simulink model "Model_6DOF_2021a"  (R2021b)
settings: Solver=FixedStepAuto  StartTime=0.0  StopTime=Tfin  FixedStep=0.05  RelTol=1e-3
values from neighbouring files (symbols this model uses):
  adap = 1    [ctrl_mode_param.m]
  Ba_0 = [0 0 0 0 0 0]    [ctrl_mode_param.m]
  Bv_0 = [tgt_speed 0 0 0 0 0]    [ctrl_mode_param.m]
  Bx_0 = [0 0 tgt_depth 0 0 0]    [ctrl_mode_param.m]
  check_angle = 10    [ctrl_mode_param.m]
  Cp = [Cpx' ; Cpy' ; Cpz']    [ctrl_mode_param.m]
  Cp_prime = Cp*Dm    [ctrl_mode_param.m]
  ctrl_mode = 5    [run.m]
  dX_imposed = 10    [ctrl_mode_param.m]
  Seastate = 5    [ctrl_mode_param.m]    (also in run.m = 0)
  tgt_depth = -50    [ctrl_mode_param.m]
  tgt_pitch = 0    [ctrl_mode_param.m]
  tgt_speed = -5    [ctrl_mode_param.m]
  tgt_sway = 0    [ctrl_mode_param.m]
  tgt_yaw = 0    [ctrl_mode_param.m]
undefined symbols (not defined in the file or in its folder): Bb, dA_BP1, dA_BP2, dA_Hull, dA_PH, dA_Sail, dA_SProot, dA_X1a, dA_X1b, dA_X2a, dA_X2b, dA_X3a, dA_X3b, dA_X4a, dA_X4b, Ixx, Ixy, Ixz, Iyy, Iyz, Izz, Mb, n_BP1, n_BP2, n_Hull, n_PH, n_Sail, n_SProot, n_X2a, n_X2b, n_X3a, n_X4a, n_X4b, nt_BP1, nt_BP2, nt_Hull, nt_PH, nt_Sail, nt_SProot, nt_X1a, nt_X1b, nt_X2a, nt_X2b, nt_X3a, nt_X3b, nt_X4a, nt_X4b, vt1_BP1, vt1_BP2, vt1_Hull, vt1_PH, vt1_Sail, vt1_SProot, vt1_X1a, vt1_X1b, vt1_X2a, vt1_X2b, vt1_X3a, vt1_X3b, vt1_X4a ... (+36)
libraries: simulink x19
(part 1 of 6)
settings Model: Creator=yagkim  LastModifiedBy=vcichella_l
settings SolverCC: AlgebraicLoopSolver=TrustRegion
settings DebuggingCC: SFMachineParentedDataDiag=warning  ArithmeticOperatorsInVariantConditions=warning
settings SFSimCC: CustomCodeUndefinedFunction=UseInterfaceOnly

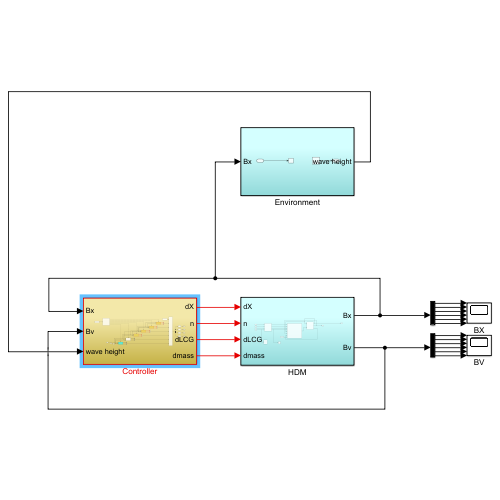
[thumbnail: Simulink's stored preview of the top-level diagram]
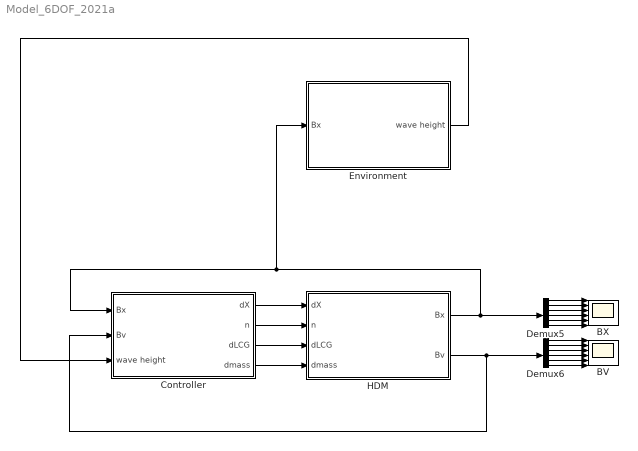
== system Model_6DOF_2021a ==
  BV : Scope  NumInputPorts=6
  BX : Scope  NumInputPorts=6
  Controller : Subsystem
  Demux5 : Demux  Outputs=6
  Demux6 : Demux  Outputs=6
  Environment : Subsystem
  HDM : Subsystem
  wires:
  HDM/1(Bx) -> Environment/1(Bx), Controller/1(Bx), Demux5/1
  Demux6/4 -> BV/4
  HDM/2(Bv) -> Demux6/1, Controller/2(Bv)
  Demux6/6 -> BV/6
  Demux5/5 -> BX/5
  Demux6/2 -> BV/2
  Demux5/6 -> BX/6
  Demux6/5 -> BV/5
  Demux5/4 -> BX/4
  Demux6/1 -> BV/1
  Demux5/3 -> BX/3
  Demux6/3 -> BV/3
  Demux5/2 -> BX/2
  Demux5/1 -> BX/1
  Controller/1(dX) -> HDM/1(dX)
  Controller/2(n) -> HDM/2(n)
  Controller/3(dLCG) -> HDM/3(dLCG)
  Controller/4(dmass) -> HDM/4(dmass)
  Environment/1(wave height) -> Controller/3(wave height)

== system Model_6DOF_2021a/Controller ==
  Bx : Inport
  Bv : Inport  Port=2
  wave height : Inport  Port=3
  Constant : Constant  Value=ctrl_mode
  Constant1 : Constant  Value=ctrl_mode
  HZZ : Subsystem  TreatAsAtomicUnit=on
  Multiport Switch : MultiPortSwitch  Inputs=6
  Mux{,1..5} (6 alike) : Mux
  PF+L1 : Subsystem  TreatAsAtomicUnit=on
  SP : Subsystem  TreatAsAtomicUnit=on
  Selector : Selector  InputPortWidth=8  IndexOptions=Index vector (dialog)  Indices=[1 2 3 4 5]  OutputSizes=1
  Selector1 : Selector  InputPortWidth=8  IndexOptions=Index vector (dialog)  Indices=7  OutputSizes=1
  Selector2 : Selector  InputPortWidth=8  IndexOptions=Index vector (dialog)  Indices=8  OutputSizes=1
  Selector3 : Selector  InputPortWidth=8  IndexOptions=Index vector (dialog)  Indices=6  OutputSizes=1
  Switch Case : SwitchCase  CaseConditions={1,2,3,4,5}
  TC : Subsystem  TreatAsAtomicUnit=on
  VZZ : Subsystem  TreatAsAtomicUnit=on
  customize : Subsystem  TreatAsAtomicUnit=on
  dX : Outport  VectorParamsAs1DForOutWhenUnconnected=off
  n : Outport  Port=2  VectorParamsAs1DForOutWhenUnconnected=off
  dLCG : Outport  Port=3  VectorParamsAs1DForOutWhenUnconnected=off
  dmass : Outport  Port=4  VectorParamsAs1DForOutWhenUnconnected=off
  wires:
  Constant/1 -> Switch Case/1
  Switch Case/1 -> HZZ/Action
  Switch Case/2 -> SP/Action
  Switch Case/3 -> TC/Action
  Switch Case/4 -> VZZ/Action
  Multiport Switch/1 -> Selector3/1, Selector2/1, Selector1/1, Selector/1
  Selector/1 -> dX/1
  Selector3/1 -> n/1
  Selector2/1 -> dmass/1
  Selector1/1 -> dLCG/1
  Bx/1 -> customize/1(Bx), PF+L1/1(Bx), VZZ/1(Bx), HZZ/1(Bx), SP/1(Bx), TC/1(Bx)
  Bv/1 -> customize/2(Bv), PF+L1/2(Bv), VZZ/2(Bv), HZZ/2(Bv), SP/2(Bv), TC/2(Bv)
  HZZ/1(dX) -> Mux/1
  HZZ/2(n) -> Mux/2
  HZZ/3(dLCG) -> Mux/3
  HZZ/4(dmass) -> Mux/4
  SP/1(dX) -> Mux1/1
  SP/2(n) -> Mux1/2
  SP/3(dLCG) -> Mux1/3
  SP/4(dmass) -> Mux1/4
  Mux1/1 -> Multiport Switch/3
  TC/1(dX) -> Mux2/1
  TC/2(n) -> Mux2/2
  TC/3(dLCG) -> Mux2/3
  TC/4(dmass) -> Mux2/4
  VZZ/1(dX) -> Mux3/1
  VZZ/2(n) -> Mux3/2
  VZZ/3(dLCG) -> Mux3/3
  VZZ/4(dmass) -> Mux3/4
  PF+L1/1(dX) -> Mux4/1
  PF+L1/2(n) -> Mux4/2
  PF+L1/3(dLCG) -> Mux4/3
  PF+L1/4(dmass) -> Mux4/4
  Switch Case/5 -> PF+L1/Action
  customize/4(dmass) -> Mux5/4
  customize/3(dLCG) -> Mux5/3
  customize/2(n) -> Mux5/2
  customize/1(dX) -> Mux5/1
  Switch Case/6 -> customize/Action
  wave height/1 -> PF+L1/3(wave height), SP/3(wave height), TC/3(wave height), customize/3(wave height)
  Mux/1 -> Multiport Switch/2
  Mux2/1 -> Multiport Switch/4
  Mux3/1 -> Multiport Switch/5
  Mux4/1 -> Multiport Switch/6
  Mux5/1 -> Multiport Switch/7
  Constant1/1 -> Multiport Switch/1

== system Model_6DOF_2021a/Environment ==
  Bx : Inport
  Constant : Constant  Value=0
  Terminator : Terminator
  wave height : Outport
  wires:
  Bx/1 -> Terminator/1
  Constant/1 -> wave height/1

== system Model_6DOF_2021a/HDM ==
  dX : Inport
  n : Inport  Port=2
  dLCG : Inport  Port=3
  dmass : Inport  Port=4
  Constant1 : Constant  Value=Seastate
  HDM B3 : Subsystem  InitFcn='main'
  Integration and Coord. Transfrom : Subsystem
  Scope : Scope
  Scope1 : Scope
  actuator saturation : Subsystem
  Bx : Outport
  Bv : Outport  Port=2
  wires:
  Integration and Coord. Transfrom/3(Ba) -> HDM B3/7(Ba)
  Integration and Coord. Transfrom/2(Bv) -> Bv/1, HDM B3/6(Bv)
  HDM B3/1(F_hyd) -> Integration and Coord. Transfrom/2(F_hyd)
  Constant1/1 -> HDM B3/8(SeaState)
  Integration and Coord. Transfrom/1("Bx ") -> Bx/1, Integration and Coord. Transfrom/1(Bx), HDM B3/5(Bx)
  dX/1 -> actuator saturation/1("dX ")
  n/1 -> actuator saturation/2("n ")
  dLCG/1 -> actuator saturation/3(dLCG)
  dmass/1 -> Scope/1, actuator saturation/4(dmass)
  actuator saturation/1(dX) -> HDM B3/1(dX CTRL)
  actuator saturation/2(n) -> HDM B3/2(n)
  actuator saturation/3(dLCG (m)) -> HDM B3/3(dLCG)
  actuator saturation/4(dmass (kg)) -> Scope1/1, HDM B3/4(dmass)

== system Model_6DOF_2021a/Controller/HZZ ==
  note: SbDn
  note: SbUp
  note: PsDn
  note: Sail
  note: PsUp
  Bx : Inport
  Bv : Inport  Port=2
  Action Port : ActionPort  ActionPortLabel=case [ 1 ]:
  Add3 : Sum  Inputs=+-
  Add4 : Sum
  Add5 : Sum  Inputs=-+
  Add6 : Sum  Inputs=--
  Constant : Constant  Value=0
  Constant1 : Constant  Value=0
  Constant2 : Constant  Value=tgt_depth
  Gain : Gain  Gain=-1/4
  Gain1 : Gain  Gain=-1
  Mux : Mux  Inputs=5
  Subsystem : Subsystem
  Target Pitch : Constant  Value=tgt_pitch
  Target Speed2 : Constant  Value=tgt_speed
  Terminator : Terminator
  dV PID : Subsystem
  dX : Outport
  n : Outport  Port=2
  dLCG : Outport  Port=3
  dmass : Outport  Port=4
  wires:
  Gain1/1 -> Mux/5
  Add6/1 -> Mux/4
  dV PID/1(dV_pid) -> Add3/1, Add4/1, Add5/1, Add6/1, Gain1/1
  Add4/1 -> Mux/2
  Add3/1 -> Mux/1
  Add5/1 -> Mux/3
  Bx/1 -> dV PID/1(Bx), Subsystem/1(Bx)
  Mux/1 -> dX/1  "dX"
  Target Pitch/1 -> dV PID/2(Target Pitch)
  Constant2/1 -> dV PID/3(Target Height)
  Constant/1 -> dmass/1
  Constant1/1 -> dLCG/1
  Target Speed2/1 -> Gain/1
  Gain/1 -> n/1
  Subsystem/1(dH_HZZ) -> Add3/2, Add6/2, Add5/2, Add4/2
  Bv/1 -> Terminator/1

== system Model_6DOF_2021a/Controller/PF+L1 ==
  Bx : Inport
  Bv : Inport  Port=2
  wave height : Inport  Port=3
  Action Port : ActionPort  ActionPortLabel=case [ 5 ]:
  Constant1 : Constant  Value=0
  Constant2 : Constant  Value=tgt_speed
  Constant3 : Constant  Value=adap
  Scope : Scope
  Stop Simulation : Stop
  Terminator2 : Terminator
  pf_controller : MATLAB Function  TreatAsAtomicUnit=on
  dX : Outport
  n : Outport  Port=2
  dLCG : Outport  Port=3
  dmass : Outport  Port=4
  wires:
  Constant1/1 -> dmass/1, dLCG/1
  wave height/1 -> Terminator2/1
  pf_controller/1(dX) -> dX/1
  pf_controller/2(n) -> n/1
  pf_controller/3(stop) -> Stop Simulation/1
  Constant2/1 -> pf_controller/3(ref)
  Constant3/1 -> pf_controller/4(adap)
  pf_controller/4(pd) -> Scope/1
  Bv/1 -> pf_controller/1(Bv)
  Bx/1 -> pf_controller/2(Bx)

== system Model_6DOF_2021a/Controller/SP ==
  note: PsUp
  note: Sail
  note: PsDn
  note: SbUp
  note: SbDn
  Bx : Inport
  Bv : Inport  Port=2
  wave height : Inport  Port=3
  Action Port : ActionPort  ActionPortLabel=case [ 2 ]:
  " " : Constant  Value=tgt_sway
  "  " : Constant  Value=tgt_yaw
  Add3 : Sum  Inputs=+-
  Add4 : Sum
  Add5 : Sum  Inputs=-+
  Add6 : Sum  Inputs=--
  "Bx " : InportShadow
  Constant : Constant  Value=0
  Gain : Gain  Gain=-1
  Mux : Mux  Inputs=5
  Selector : Selector  InputPortWidth=6  IndexOptions=Index vector (dialog)  Indices=3  OutputSizes=1
  Sum : Sum  Inputs=|+-
  Target Depth2 : Constant  Value=tgt_depth
  Target Height : Constant  Value=tgt_depth
  Target Pitch1 : Constant  Value=tgt_pitch
  Target Pitch2 : Constant  Value=tgt_pitch
  Target Speed1 : Constant  Value=tgt_speed
  Trim and Ballast Tank PID : Subsystem
  dH PID : Subsystem
  dV PID : Subsystem
  n:RPS PID : Subsystem
  dX : Outport
  n : Outport  Port=2
  dLCG : Outport  Port=3
  dmass : Outport  Port=4
  wires:
  n:RPS PID/1(n_ctrl) -> n/1
  Gain/1 -> Mux/5
  Target Speed1/1 -> n:RPS PID/1(Target Speed)
  Target Height/1 -> Trim and Ballast Tank PID/3(Target Height)
  Target Pitch1/1 -> Trim and Ballast Tank PID/2(Target Pitch)
  Mux/1 -> dX/1  "dX"
  "  "/1 -> dH PID/1(Target Yaw)
  " "/1 -> dH PID/2(Target Sway)
  dH PID/1(dH_PID) -> Add4/2, Add6/2, Add5/2, Add3/2
  Bv/1 -> n:RPS PID/2(Bv)
  Add5/1 -> Mux/3
  Add3/1 -> Mux/1
  Add4/1 -> Mux/2
  Add6/1 -> Mux/4
  Constant/1 -> dLCG/1
  "Bx "/1 -> Trim and Ballast Tank PID/1(Bx)
  Selector/1 -> Sum/1  "current"
  Bx/1 -> dH PID/3(Bx), dV PID/1(Bx), Selector/1
  Target Depth2/1 -> dV PID/3(Target Height)
  Target Pitch2/1 -> dV PID/2(Target Pitch)
  dV PID/1(dV_pid) -> Add6/1, Add5/1, Add4/1, Add3/1, Gain/1
  Trim and Ballast Tank PID/2(dmass) -> dmass/1
  wave height/1 -> Sum/2
  Sum/1 -> dV PID/4(Zeff)

== system Model_6DOF_2021a/Controller/TC ==
  note: SbDn
  note: SbUp
  note: PsDn
  note: Sail
  note: PsUp
  Bx : Inport
  Bv : Inport  Port=2
  wave height : Inport  Port=3
  Action Port : ActionPort  ActionPortLabel=case [ 3 ]:
  Add3 : Sum  Inputs=+-
  Add4 : Sum
  Add5 : Sum  Inputs=-+
  Add6 : Sum  Inputs=--
  Bx1 : InportShadow
  Constant : Constant  Value=dX_imposed
  Constant1 : Constant  Value=0
  Gain : Gain  Gain=-1
  Mux : Mux  Inputs=5
  Selector : Selector  InputPortWidth=6  IndexOptions=Index vector (dialog)  Indices=3  OutputSizes=1
  Sum : Sum  Inputs=|+-
  Target Depth1 : Constant  Value=tgt_depth
  Target Height : Constant  Value=tgt_depth
  Target Pitch : Constant  Value=tgt_pitch
  Target Pitch1 : Constant  Value=tgt_pitch
  Target Speed1 : Constant  Value=tgt_speed
  Trim and Ballast Tank PID : Subsystem
  dV PID : Subsystem
  n:RPS PID : Subsystem
  dX : Outport
  n : Outport  Port=2
  dLCG : Outport  Port=3
  dmass : Outport  Port=4
  wires:
  Gain/1 -> Mux/5
  Add6/1 -> Mux/4
  dV PID/1(dV_pid) -> Add3/1, Add4/1, Add5/1, Add6/1, Gain/1
  Add4/1 -> Mux/2
  Add3/1 -> Mux/1
  Add5/1 -> Mux/3
  Bv/1 -> n:RPS PID/2(Bv)
  Mux/1 -> dX/1  "dX"
  n:RPS PID/1(n_ctrl) -> n/1
  Target Pitch/1 -> dV PID/2(Target Pitch)
  Target Speed1/1 -> n:RPS PID/1(Target Speed)
  Target Depth1/1 -> dV PID/3(Target Height)
  Constant/1 -> Add6/2, Add5/2, Add4/2, Add3/2
  Constant1/1 -> dLCG/1
  Trim and Ballast Tank PID/2(dmass) -> dmass/1
  Target Pitch1/1 -> Trim and Ballast Tank PID/2(Target Pitch)
  Target Height/1 -> Trim and Ballast Tank PID/3(Target Height)
  Bx1/1 -> Trim and Ballast Tank PID/1(Bx)
  Selector/1 -> Sum/1  "current"
  Bx/1 -> Selector/1, dV PID/1(Bx)
  wave height/1 -> Sum/2
  Sum/1 -> dV PID/4(Zeff)

== system Model_6DOF_2021a/Controller/VZZ ==
  note: PsUp
  note: Sail
  note: PsDn
  note: SbUp
  note: SbDn
  Bx : Inport
  Bv : Inport  Port=2
  Action Port : ActionPort  ActionPortLabel=case [ 4 ]:
  " " : Constant  Value=tgt_sway
  "  " : Constant  Value=tgt_yaw
  Add3 : Sum  Inputs=+-
  Add4 : Sum
  Add5 : Sum  Inputs=-+
  Add6 : Sum  Inputs=--
  Constant : Constant  Value=0
  Constant1 : Constant  Value=0
  Constant2 : Constant  Value=0
  Gain : Gain  Gain=-1/4
  Gain2 : Gain  Gain=-1
  Mux : Mux  Inputs=5
  Scope : Scope
  Target Speed2 : Constant  Value=tgt_speed
  Terminator : Terminator
  dH PID : Subsystem
  dV : Subsystem
  dX : Outport
  n : Outport  Port=2
  dLCG : Outport  Port=3
  dmass : Outport  Port=4
  wires:
  Gain2/1 -> Mux/5
  Mux/1 -> dX/1  "dX"
  "  "/1 -> dH PID/1(Target Yaw)
  " "/1 -> dH PID/2(Target Sway)
  dH PID/1(dH_PID) -> Add4/2, Add6/2, Add5/2, Add3/2
  Bx/1 -> dH PID/3(Bx), dV/1(Bx)
  Add5/1 -> Mux/3
  Add3/1 -> Mux/1
  Add4/1 -> Mux/2
  Add6/1 -> Mux/4
  Target Speed2/1 -> Gain/1
  Gain/1 -> n/1
  Constant1/1 -> dLCG/1
  Constant/1 -> dmass/1
  dV/1(dV_VZZ) -> Scope/1, Add6/1, Add5/1, Add4/1, Add3/1
  Bv/1 -> Terminator/1
  Constant2/1 -> Gain2/1

== system Model_6DOF_2021a/Controller/customize ==
  Bx : Inport
  Bv : Inport  Port=2
  wave height : Inport  Port=3
  Action Port : ActionPort  ActionPortLabel=default:
  Constant : Constant  Value=zeros(5,1)
  Constant1 : Constant  Value=0
  Terminator : Terminator
  Terminator1 : Terminator
  Terminator2 : Terminator
  dX : Outport
  n : Outport  Port=2
  dLCG : Outport  Port=3
  dmass : Outport  Port=4
  wires:
  Constant1/1 -> dmass/1, n/1, dLCG/1
  Constant/1 -> dX/1
  Bv/1 -> Terminator1/1
  Bx/1 -> Terminator/1
  wave height/1 -> Terminator2/1

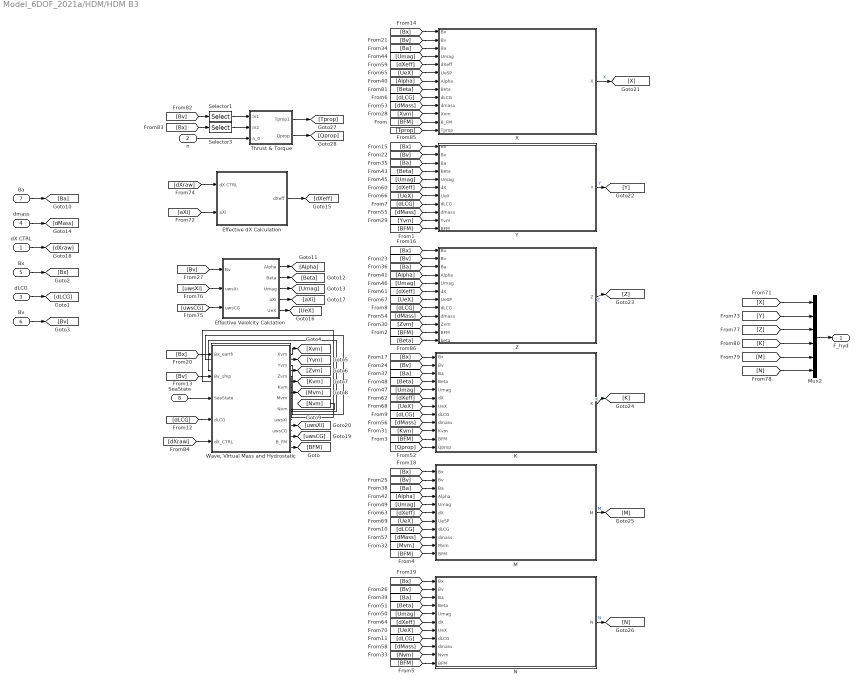
== system Model_6DOF_2021a/HDM/HDM B3 ==
  dX CTRL : Inport
  n : Inport  Port=2
  dLCG : Inport  Port=3
  dmass : Inport  Port=4
  Bx : Inport  Port=5
  Bv : Inport  Port=6
  Ba : Inport  Port=7
  SeaState : Inport  Port=8
  Effective Veloicity Calclation : Subsystem
  Effective dX Calculation : Subsystem
  K : Subsystem
  M : Subsystem
  Mux2 : Mux  Inputs=6
  N : Subsystem
  Selector1 : Selector  InputPortWidth=6  IndexOptions=Index vector (dialog)  Indices=1  OutputSizes=1
  Selector3 : Selector  InputPortWidth=6  IndexOptions=Index vector (dialog)  Indices=3  OutputSizes=1
  Thrust & Torque : Subsystem
  "Wave, Virtual Mass and Hydrostatic" : Subsystem
  X : Subsystem
  Y : Subsystem
  Z : Subsystem
  F_hyd : Outport  VectorParamsAs1DForOutWhenUnconnected=off
  wires:
  Mux2/1 -> F_hyd/1
  Effective dX Calculation/1(dXeff) -> [dXeff]
  Ba/1 -> [Ba]
  Bx/1 -> [Bx]
  dLCG/1 -> [dLCG]
  Bv/1 -> [Bv]
  SeaState/1 -> "Wave, Virtual Mass and Hydrostatic"/3(SeaState)
  n/1 -> Thrust & Torque/3(n_0)
  "Wave, Virtual Mass and Hydrostatic"/9(B_FM) -> [BFM]
  [BFM] -> X/12(B_FM)
  [BFM] -> Y/11(BFM)
  [BFM] -> Z/11(BFM)
  [BFM] -> K/11(BFM)
  [BFM] -> M/11(BFM)
  [BFM] -> N/11(BFM)
  [dLCG] -> X/9(dLCG)
  [dLCG] -> Y/8(dLCG)
  [dLCG] -> Z/8(dLCG)
  [dLCG] -> K/8(dLCG)
  [dLCG] -> M/8(dLCG)
  [dLCG] -> N/8(dLCG)
  [dLCG] -> "Wave, Virtual Mass and Hydrostatic"/4(dLCG)
  [Bx] -> X/1(Bx)
  [Bx] -> Y/1(Bx)
  [Bx] -> Z/1(Bx)
  [Bx] -> K/1(Bx)
  [Bx] -> M/1(Bx)
  [Bx] -> N/1(Bx)
  [Bx] -> "Wave, Virtual Mass and Hydrostatic"/1(Bx_earth)
  [Bv] -> "Wave, Virtual Mass and Hydrostatic"/2(Bv_ship)
  [Bv] -> X/2(Bv)
  [Bv] -> Y/2(Bv)
  [Bv] -> K/2(Bv)
  [Bv] -> M/2(Bv)
  [Bv] -> N/2(Bv)
  [Bv] -> Effective Veloicity Calclation/1(Bv)
  "Wave, Virtual Mass and Hydrostatic"/1(Xvm) -> [Xvm]
  "Wave, Virtual Mass and Hydrostatic"/2(Yvm) -> [Yvm]
  "Wave, Virtual Mass and Hydrostatic"/3(Zvm) -> [Zvm]
  "Wave, Virtual Mass and Hydrostatic"/4(Kvm) -> [Kvm]
  "Wave, Virtual Mass and Hydrostatic"/5(Mvm) -> [Mvm]
  "Wave, Virtual Mass and Hydrostatic"/6(Nvm) -> [Nvm]
  [Xvm] -> X/11(Xvm)
  [Yvm] -> Y/10(Yvm)
  [Zvm] -> Z/10(Zvm)
  [Bv] -> Z/2(Bv)
  [Kvm] -> K/10(Kvm)
  [Mvm] -> M/10(Mvm)
  [Nvm] -> N/10(Nvm)
  [Ba] -> X/3(Ba)
  [Ba] -> Y/3(Ba)
  [Ba] -> Z/3(Ba)
  [Ba] -> K/3(Ba)
  [Ba] -> M/3(Ba)
  [Ba] -> N/3(Ba)
  Effective Veloicity Calclation/1(Alpha) -> [Alpha]
  [Alpha] -> X/7(Alpha)
  [Alpha] -> Z/4(Alpha)
  [Alpha] -> M/4(Alpha)
  Effective Veloicity Calclation/2(Beta) -> [Beta]
  [Beta] -> Y/4(Beta)
  Effective Veloicity Calclation/3(Umag) -> [Umag]
  [Umag] -> X/4(Umag)
  [Umag] -> Y/5(Umag)
  [Umag] -> Z/5(Umag)
  [Umag] -> K/5(Umag)
  [Beta] -> K/4(Beta)
  [Umag] -> M/5(Umag)
  [Umag] -> N/5(Umag)
  [Beta] -> N/4(Beta)
  dmass/1 -> [dMass]
  [dMass] -> X/10(dmass)
  [dMass] -> Z/9(dmass)
  [dMass] -> Y/9(dmass)
  [dMass] -> K/9(dmass)
  [dMass] -> M/9(dmass)
  [dMass] -> N/9(dmass)
  [dXeff] -> X/5(dXeff)
  [dXeff] -> Y/6(dX)
  [dXeff] -> Z/6(dX)
  [dXeff] -> K/6(dX)
  [dXeff] -> M/6(dX)
  [dXeff] -> N/6(dX)
  Effective Veloicity Calclation/5(UeX) -> [UeX]
  [UeX] -> X/6(UeSP)
  [UeX] -> Y/7(UeX)
  [UeX] -> Z/7(UeSP)
  [UeX] -> K/7(UeX)
  [UeX] -> M/7(UeSP)
  [UeX] -> N/7(UeX)
  Effective Veloicity Calclation/4(aXi) -> [aXi]
  [aXi] -> Effective dX Calculation/2(aXi)
  dX CTRL/1 -> [dXraw]
  [dXraw] -> Effective dX Calculation/1(dX CTRL)
  "Wave, Virtual Mass and Hydrostatic"/8(uwsCG) -> [uwsCG]
  [uwsCG] -> Effective Veloicity Calclation/3(uwsCG)
  "Wave, Virtual Mass and Hydrostatic"/7(uwsXi) -> [uwsXi]
  [uwsXi] -> Effective Veloicity Calclation/2(uwsXi)
  X/1(X) -> [X]  "X"
  Y/1(Y) -> [Y]  "Y"
  Z/1(Z) -> [Z]  "Z"
  K/1(K) -> [K]  "K"
  M/1(M) -> [M]  "M"
  N/1(N) -> [N]  "N"
  [Beta] -> X/8(Beta)
  [dXraw] -> "Wave, Virtual Mass and Hydrostatic"/5(dX_CTRL)
  [X] -> Mux2/1
  [Y] -> Mux2/2
  [Z] -> Mux2/3
  [K] -> Mux2/4
  [M] -> Mux2/5
  [N] -> Mux2/6
  [Qprop] -> K/12(Qprop)
  [Bv] -> Selector1/1
  Selector1/1 -> Thrust & Torque/1(In1)
  Selector3/1 -> Thrust & Torque/2(In2)
  [Bx] -> Selector3/1
  Thrust & Torque/1(Tprop1) -> [Tprop]
  [Tprop] -> X/13(Tprop)
  Thrust & Torque/2(Qprop) -> [Qprop]
  [Beta] -> Z/12(beta)

== system Model_6DOF_2021a/HDM/Integration and Coord. Transfrom ==
  Bx : Inport
  F_hyd : Inport  Port=2
  Coordinate Transform : Subsystem
  Rigid Body Motion : Subsystem
  "Bx " : Outport
  Bv : Outport  Port=2
  Ba : Outport  Port=3
  wires:
  Coordinate Transform/1(X_earth) -> "Bx "/1
  Rigid Body Motion/1(Bv) -> Bv/1, Coordinate Transform/1(Bv)
  Rigid Body Motion/2(Ba) -> Ba/1
  F_hyd/1 -> Rigid Body Motion/1(F_hyd)
  Bx/1 -> Rigid Body Motion/2(Bx)

== system Model_6DOF_2021a/HDM/actuator saturation ==
  "dX " : Inport
  "n " : Inport  Port=2
  dLCG : Inport  Port=3
  dmass : Inport  Port=4
  " " : Subsystem
  "   " : Subsystem
  Subsystem1 : Subsystem
  Subsystem2 : Subsystem
  dX : Outport
  n : Outport  Port=2
  dLCG (m) : Outport  Port=3
  dmass (kg) : Outport  Port=4
  wires:
  "   "/1(n) -> n/1
  " "/1(dX) -> dX/1
  dLCG/1 -> Subsystem1/1(dLCG)
  Subsystem1/1(dLCG (m)) -> dLCG (m)/1
  dmass/1 -> Subsystem2/1(dmass)
  "dX "/1 -> " "/1("dX ")
  Subsystem2/1(dmass (kg)) -> dmass (kg)/1
  "n "/1 -> "   "/1("n ")

== system Model_6DOF_2021a/Controller/HZZ/Subsystem ==
  Bx : Inport
  Clock : Clock
  Constant4 : Constant  Value=dX_imposed
  Constant6 : Constant  Value=check_angle
  Gain1 : Gain  Gain=-1
  Gain10 : Gain  Gain=180/pi
  Integrator2 : Integrator
  MATLAB Function : MATLAB Function  TreatAsAtomicUnit=on
  Max Fin Rate : Constant  Value=7.11
  Saturation1 : Saturate  UpperLimit=20  LowerLimit=-20
  Selector3 : Selector  InputPortWidth=6  IndexOptions=Index vector (dialog)  Indices=6  OutputSizes=1
  dH_HZZ : Outport
  wires:
  Saturation1/1 -> MATLAB Function/4(dVprev), Gain1/1
  Bx/1 -> Selector3/1
  Selector3/1 -> Gain10/1
  Max Fin Rate/1 -> MATLAB Function/1(rate)
  Clock/1 -> MATLAB Function/2(trigger)
  Gain10/1 -> MATLAB Function/3(X5)
  MATLAB Function/1(dVrate) -> Integrator2/1
  Integrator2/1 -> Saturation1/1
  Constant6/1 -> MATLAB Function/6(dXmax)
  Constant4/1 -> MATLAB Function/5(dVmax)
  Gain1/1 -> dH_HZZ/1

== system Model_6DOF_2021a/Controller/HZZ/dV PID ==
  Bx : Inport
  Target Pitch : Inport  Port=2
  Target Height : Inport  Port=3
  Add : Sum  Inputs=+++
  Add1 : Sum  Inputs=+++
  Add10 : Sum
  Add7 : Sum  Inputs=-+
  Add9 : Sum  Inputs=-+
  Constant : Constant  Value=7.11
  Constant1 : Constant  Value=-7.11
  D-Depth : Gain  Gain=3
  D-Pitch : Gain  Gain=3
  Derivative : Derivative
  Derivative3 : Derivative
  Gain36 : Gain  Gain=180/pi
  I-Depth : Gain  Gain=0.1044
  I-Pitch : Gain  Gain=0.1466
  I-Pitch{1..6} (6 alike) : Gain
  Integrator : Integrator
  Integrator3 : Integrator
  Max Deflection1 : Saturate  UpperLimit=30  LowerLimit=-30
  P-Depth : Gain  Gain=3
  P-Pitch : Gain  Gain=3
  PID Pitch : Selector  InputPortWidth=6  IndexOptions=Index vector (dialog)  Indices=5  OutputSizes=1
  PID Pitch1 : Selector  InputPortWidth=6  IndexOptions=Index vector (dialog)  Indices=3  OutputSizes=1
  Rate Limiter Dynamic : simulink/Discontinuities/Rate Limiter Dynamic
  dV_pid : Outport
  wires:
  Max Deflection1/1 -> dV_pid/1  "dV"
  Add/1 -> Add10/2  "dV Depth (deg)"
  Add7/1 -> Derivative3/1, Integrator/1, P-Depth/1  "Erorr in z (m)"
  PID Pitch1/1 -> Add7/2  "z (m)"
  Integrator/1 -> I-Depth/1
  P-Depth/1 -> I-Pitch4/1
  Gain36/1 -> Add9/2  "Pitch (deg)"
  Add9/1 -> Derivative/1, Integrator3/1, P-Pitch/1  "Error in Pitch (deg)"
  P-Pitch/1 -> I-Pitch3/1
  Bx/1 -> PID Pitch1/1, PID Pitch/1
  Derivative3/1 -> D-Depth/1
  Add1/1 -> Add10/1  "dV Pitch (deg)"
  D-Depth/1 -> I-Pitch6/1
  Derivative/1 -> D-Pitch/1
  Integrator3/1 -> I-Pitch/1
  PID Pitch/1 -> Gain36/1
  Rate Limiter Dynamic/1 -> Max Deflection1/1  "dV"
  D-Pitch/1 -> I-Pitch5/1
  Target Pitch/1 -> Add9/1
  Add10/1 -> Rate Limiter Dynamic/2
  Constant/1 -> Rate Limiter Dynamic/1
  Constant1/1 -> Rate Limiter Dynamic/3
  Target Height/1 -> Add7/1
  I-Pitch/1 -> I-Pitch1/1
  I-Depth/1 -> I-Pitch2/1
  I-Pitch1/1 -> Add1/2
  I-Pitch2/1 -> Add/2
  I-Pitch3/1 -> Add1/1
  I-Pitch4/1 -> Add/1
  I-Pitch5/1 -> Add1/3
  I-Pitch6/1 -> Add/3

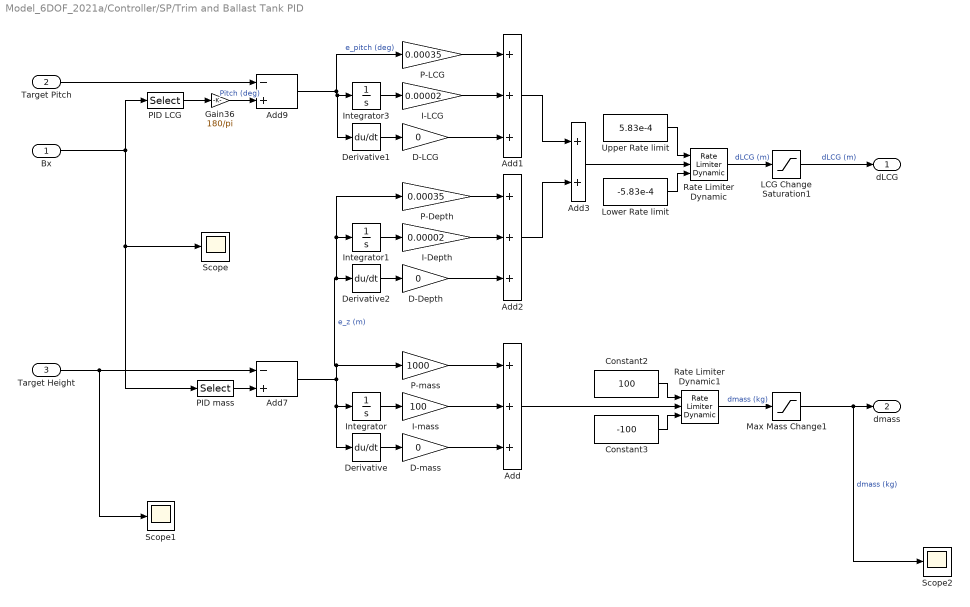
== system Model_6DOF_2021a/Controller/SP/Trim and Ballast Tank PID ==
  Bx : Inport
  Target Pitch : Inport  Port=2
  Target Height : Inport  Port=3
  " LCG Change Saturation1" : Saturate
  Add : Sum  Inputs=+++
  Add1 : Sum  Inputs=+++
  Add2 : Sum  Inputs=+++
  Add3 : Sum
  Add7 : Sum  Inputs=-+
  Add9 : Sum  Inputs=-+
  Constant2 : Constant  Value=100
  Constant3 : Constant  Value=-100
  D-Depth : Gain  Gain=0
  D-LCG : Gain  Gain=0
  D-mass : Gain  Gain=0
  Derivative : Derivative
  Derivative1 : Derivative
  Derivative2 : Derivative
  Gain36 : Gain  Gain=180/pi
  I-Depth : Gain  Gain=0.00002
  I-LCG : Gain  Gain=0.00002
  I-mass : Gain  Gain=100
  Integrator : Integrator
  Integrator1 : Integrator
  Integrator3 : Integrator
  Lower Rate limit : Constant  Value=-5.83e-4
  Max Mass Change1 : Saturate  UpperLimit=20000  LowerLimit=-20000
  P-Depth : Gain  Gain=0.00035
  P-LCG : Gain  Gain=0.00035
  P-mass : Gain  Gain=1000
  PID LCG : Selector  InputPortWidth=6  IndexOptions=Index vector (dialog)  Indices=5  OutputSizes=1
  PID mass : Selector  InputPortWidth=6  IndexOptions=Index vector (dialog)  Indices=3  OutputSizes=1
  Rate Limiter Dynamic : simulink/Discontinuities/Rate Limiter Dynamic
  Rate Limiter Dynamic1 : simulink/Discontinuities/Rate Limiter Dynamic
  Scope : Scope
  Scope1 : Scope
  Scope2 : Scope
  Upper Rate limit : Constant  Value=5.83e-4
  dLCG : Outport
  dmass : Outport  Port=2
  wires:
  " LCG Change Saturation1"/1 -> dLCG/1  "dLCG (m)"
  Max Mass Change1/1 -> Scope2/1, dmass/1  "dmass (kg)"
  Add9/1 -> P-LCG/1, Integrator3/1, Derivative1/1  "e_pitch (deg)"
  Add7/1 -> P-mass/1, Derivative2/1, Integrator1/1, P-Depth/1, Integrator/1, Derivative/1  "e_z (m)"
  Add2/1 -> Add3/2
  Add1/1 -> Add3/1
  Add3/1 -> Rate Limiter Dynamic/2
  P-Depth/1 -> Add2/1
  D-Depth/1 -> Add2/3
  Derivative2/1 -> D-Depth/1
  Integrator1/1 -> I-Depth/1
  I-Depth/1 -> Add2/2
  Constant3/1 -> Rate Limiter Dynamic1/3
  Constant2/1 -> Rate Limiter Dynamic1/1
  Add/1 -> Rate Limiter Dynamic1/2
  Rate Limiter Dynamic1/1 -> Max Mass Change1/1  "dmass (kg)"
  Lower Rate limit/1 -> Rate Limiter Dynamic/3
  Upper Rate limit/1 -> Rate Limiter Dynamic/1
  Target Pitch/1 -> Add9/1
  P-mass/1 -> Add/1
  I-LCG/1 -> Add1/2
  Integrator3/1 -> I-LCG/1
  Derivative1/1 -> D-LCG/1
  PID mass/1 -> Add7/2
  Derivative/1 -> D-mass/1
  Target Height/1 -> Scope1/1, Add7/1
  Integrator/1 -> I-mass/1
  Rate Limiter Dynamic/1 -> " LCG Change Saturation1"/1  "dLCG (m)"
  PID LCG/1 -> Gain36/1
  D-LCG/1 -> Add1/3
  P-LCG/1 -> Add1/1
  Gain36/1 -> Add9/2  "Pitch (deg)"
  I-mass/1 -> Add/2
  Bx/1 -> Scope/1, PID mass/1, PID LCG/1
  D-mass/1 -> Add/3

== system Model_6DOF_2021a/Controller/SP/dH PID ==
  Target Yaw : Inport
  Target Sway : Inport  Port=2
  Bx : Inport  Port=3
  Add1 : Sum  Inputs=+++
  Add10 : Sum
  Add2 : Sum  Inputs=+++
  Add7 : Sum  Inputs=-+
  Add9 : Sum  Inputs=-+
  Constant : Constant  Value=7.11
  Constant1 : Constant  Value=-7.11
  D-Sway : Gain  Gain=0
  D-Yaw : Gain  Gain=12.199
  Derivative : Derivative
  Derivative1 : Derivative
  Gain36 : Gain  Gain=180/pi
  I-Sway : Gain  Gain=0
  I-Yaw : Gain  Gain=0
  Integrator : Integrator
  Integrator3 : Integrator
  Max Deflection : Saturate  UpperLimit=30  LowerLimit=-30
  P-Sway1 : Gain  Gain=-1.452
  P-Yaw : Gain  Gain=3
  PID Sway : Selector  InputPortWidth=6  IndexOptions=Index vector (dialog)  Indices=2  OutputSizes=1
  PID Yaw : Selector  InputPortWidth=6  IndexOptions=Index vector (dialog)  Indices=6  OutputSizes=1
  Rate Limiter Dynamic : simulink/Discontinuities/Rate Limiter Dynamic
  dH_PID : Outport
  wires:
  Max Deflection/1 -> dH_PID/1
  Constant/1 -> Rate Limiter Dynamic/1
  Constant1/1 -> Rate Limiter Dynamic/3
  Target Yaw/1 -> Add9/1
  Add10/1 -> Rate Limiter Dynamic/2
  Derivative1/1 -> D-Yaw/1
  D-Sway/1 -> Add2/3
  P-Sway1/1 -> Add2/1
  Rate Limiter Dynamic/1 -> Max Deflection/1
  Gain36/1 -> Add9/2
  Integrator/1 -> I-Sway/1
  Add1/1 -> Add10/1
  PID Yaw/1 -> Gain36/1
  D-Yaw/1 -> Add1/3
  I-Sway/1 -> Add2/2
  Bx/1 -> PID Sway/1, PID Yaw/1
  P-Yaw/1 -> Add1/1
  PID Sway/1 -> Add7/2
  Derivative/1 -> D-Sway/1
  Target Sway/1 -> Add7/1
  Add7/1 -> Integrator/1, Derivative/1, P-Sway1/1
  I-Yaw/1 -> Add1/2
  Add2/1 -> Add10/2
  Add9/1 -> Integrator3/1, Derivative1/1, P-Yaw/1
  Integrator3/1 -> I-Yaw/1

== system Model_6DOF_2021a/Controller/SP/dV PID ==
  Bx : Inport
  Target Pitch : Inport  Port=2
  Target Height : Inport  Port=3
  Zeff : Inport  Port=4
  Add : Sum  Inputs=+++
  Add1 : Sum  Inputs=+++
  Add10 : Sum
  Add7 : Sum  Inputs=-+
  Add9 : Sum  Inputs=-+
  Constant : Constant  Value=7.11
  Constant1 : Constant  Value=-7.11
  D-Depth : Gain  Gain=3
  D-Pitch : Gain  Gain=3
  Derivative : Derivative
  Derivative3 : Derivative
  Gain36 : Gain  Gain=180/pi
  I-Depth : Gain  Gain=0.1044
  I-Pitch : Gain  Gain=0.1466
  I-Pitch{1..6} (6 alike) : Gain
  Integrator : Integrator
  Integrator3 : Integrator
  Max Deflection1 : Saturate  UpperLimit=30  LowerLimit=-30
  P-Depth : Gain  Gain=3
  P-Pitch : Gain  Gain=3
  PID Pitch : Selector  InputPortWidth=6  IndexOptions=Index vector (dialog)  Indices=5  OutputSizes=1
  Rate Limiter Dynamic : simulink/Discontinuities/Rate Limiter Dynamic
  dV_pid : Outport
  wires:
  Max Deflection1/1 -> dV_pid/1  "dV"
  Add/1 -> Add10/2  "dV Depth (deg)"
  Add7/1 -> Derivative3/1, Integrator/1, P-Depth/1  "Erorr in z (m)"
  Zeff/1 -> Add7/2  "z (m)"
  Integrator/1 -> I-Depth/1
  P-Depth/1 -> I-Pitch4/1
  Gain36/1 -> Add9/2  "Pitch (deg)"
  Add9/1 -> Derivative/1, Integrator3/1, P-Pitch/1  "Error in Pitch (deg)"
  P-Pitch/1 -> I-Pitch3/1
  Bx/1 -> PID Pitch/1
  Derivative3/1 -> D-Depth/1
  Add1/1 -> Add10/1  "dV Pitch (deg)"
  D-Depth/1 -> I-Pitch6/1
  Derivative/1 -> D-Pitch/1
  Integrator3/1 -> I-Pitch/1
  PID Pitch/1 -> Gain36/1
  Rate Limiter Dynamic/1 -> Max Deflection1/1  "dV"
  D-Pitch/1 -> I-Pitch5/1
  Target Pitch/1 -> Add9/1
  Add10/1 -> Rate Limiter Dynamic/2
  Constant/1 -> Rate Limiter Dynamic/1
  Constant1/1 -> Rate Limiter Dynamic/3
  Target Height/1 -> Add7/1
  I-Pitch/1 -> I-Pitch1/1
  I-Depth/1 -> I-Pitch2/1
  I-Pitch1/1 -> Add1/2
  I-Pitch2/1 -> Add/2
  I-Pitch3/1 -> Add1/1
  I-Pitch4/1 -> Add/1
  I-Pitch5/1 -> Add1/3
  I-Pitch6/1 -> Add/3

== system Model_6DOF_2021a/Controller/SP/n:RPS PID ==
  Target Speed : Inport
  Bv : Inport  Port=2
  Add : Sum  Inputs=+++
  Add1 : Sum  Inputs=-+
  Constant1 : Constant  Value=4
  Divide : Product  Inputs=*/
  Gain1 : Gain  Gain=14.65
  Gain4 : Gain  Gain=1.465
  Integrator : Integrator
  Rate Limiter Dynamic : simulink/Discontinuities/Rate Limiter Dynamic
  Rate Max : Constant  Value=14.65
  Rate Min : Constant  Value=-14.65
  Saturation1 : Saturate  UpperLimit=10  LowerLimit=0.01
  Selector : Selector  InputPortWidth=6  IndexOptions=Index vector (dialog)  Indices=1  OutputSizes=1
  n_ctrl : Outport  VectorParamsAs1DForOutWhenUnconnected=off
  wires:
  Saturation1/1 -> n_ctrl/1
  Rate Limiter Dynamic/1 -> Saturation1/1
  Integrator/1 -> Gain4/1
  Rate Min/1 -> Rate Limiter Dynamic/3
  Rate Max/1 -> Rate Limiter Dynamic/1
  Divide/1 -> Add/1
  Add/1 -> Rate Limiter Dynamic/2
  Gain1/1 -> Add/2
  Gain4/1 -> Add/3
  Bv/1 -> Selector/1
  Add1/1 -> Integrator/1, Gain1/1  "error term"
  Target Speed/1 -> Divide/1, Add1/1  "target"
  Constant1/1 -> Divide/2
  Selector/1 -> Add1/2  "current"

== system Model_6DOF_2021a/Controller/TC/Trim and Ballast Tank PID ==
  Bx : Inport
  Target Pitch : Inport  Port=2
  Target Height : Inport  Port=3
  " LCG Change Saturation" : Saturate
  Add : Sum  Inputs=+++
  Add1 : Sum  Inputs=+++
  Add2 : Sum  Inputs=+++
  Add3 : Sum
  Add7 : Sum  Inputs=-+
  Add9 : Sum  Inputs=-+
  Constant2 : Constant  Value=100
  Constant3 : Constant  Value=-100
  D-Depth : Gain  Gain=0
  D-LCG : Gain  Gain=0
  D-mass : Gain  Gain=0
  Derivative : Derivative
  Derivative1 : Derivative
  Derivative2 : Derivative
  Gain36 : Gain  Gain=180/pi
  I-Depth : Gain  Gain=0.00002
  I-LCG : Gain  Gain=0.00002
  I-mass : Gain  Gain=100
  Integrator : Integrator
  Integrator1 : Integrator
  Integrator3 : Integrator
  Lower Rate limit : Constant  Value=-5.83e-4
  Max Mass Change : Saturate  UpperLimit=20000  LowerLimit=-20000
  P-Depth : Gain  Gain=0.00035
  P-LCG : Gain  Gain=0.00035
  P-mass : Gain  Gain=1000
  PID LCG : Selector  InputPortWidth=6  IndexOptions=Index vector (dialog)  Indices=5  OutputSizes=1
  PID mass : Selector  InputPortWidth=6  IndexOptions=Index vector (dialog)  Indices=3  OutputSizes=1
  Rate Limiter Dynamic : simulink/Discontinuities/Rate Limiter Dynamic
  Rate Limiter Dynamic1 : simulink/Discontinuities/Rate Limiter Dynamic
  Upper Rate limit : Constant  Value=5.83e-4
  dLCG : Outport
  dmass : Outport  Port=2
  wires:
  " LCG Change Saturation"/1 -> dLCG/1  "dLCG (m)"
  Max Mass Change/1 -> dmass/1  "dmass (kg)"
  D-mass/1 -> Add/3
  Bx/1 -> PID LCG/1, PID mass/1
  I-mass/1 -> Add/2
  Gain36/1 -> Add9/2  "Pitch (deg)"
  P-LCG/1 -> Add1/1
  D-LCG/1 -> Add1/3
  PID LCG/1 -> Gain36/1
  Rate Limiter Dynamic/1 -> " LCG Change Saturation"/1
  Integrator/1 -> I-mass/1
  Target Height/1 -> Add7/1
  Derivative/1 -> D-mass/1
  PID mass/1 -> Add7/2
  Derivative1/1 -> D-LCG/1
  Integrator3/1 -> I-LCG/1
  I-LCG/1 -> Add1/2
  P-mass/1 -> Add/1
  Target Pitch/1 -> Add9/1
  Upper Rate limit/1 -> Rate Limiter Dynamic/1
  Lower Rate limit/1 -> Rate Limiter Dynamic/3
  Add/1 -> Rate Limiter Dynamic1/2
  Rate Limiter Dynamic1/1 -> Max Mass Change/1
  Constant2/1 -> Rate Limiter Dynamic1/1
  Constant3/1 -> Rate Limiter Dynamic1/3
  I-Depth/1 -> Add2/2
  Integrator1/1 -> I-Depth/1
  Derivative2/1 -> D-Depth/1
  D-Depth/1 -> Add2/3
  P-Depth/1 -> Add2/1
  Add3/1 -> Rate Limiter Dynamic/2
  Add1/1 -> Add3/1
  Add2/1 -> Add3/2
  Add7/1 -> Derivative/1, Integrator/1, P-Depth/1, Integrator1/1, Derivative2/1, P-mass/1  "e_z (m)"
  Add9/1 -> Derivative1/1, Integrator3/1, P-LCG/1  "e_pitch (deg)"

== system Model_6DOF_2021a/Controller/TC/dV PID ==
  Bx : Inport
  Target Pitch : Inport  Port=2
  Target Height : Inport  Port=3
  Zeff : Inport  Port=4
  Add : Sum  Inputs=+++
  Add1 : Sum  Inputs=+++
  Add10 : Sum
  Add7 : Sum  Inputs=-+
  Add9 : Sum  Inputs=-+
  Constant : Constant  Value=7.11
  Constant1 : Constant  Value=-7.11
  D-Depth : Gain  Gain=3
  D-Pitch : Gain  Gain=3
  Derivative : Derivative
  Derivative3 : Derivative
  Gain36 : Gain  Gain=180/pi
  I-Depth : Gain  Gain=0.1044
  I-Pitch : Gain  Gain=0.1466
  I-Pitch{1..6} (6 alike) : Gain
  Integrator : Integrator
  Integrator3 : Integrator
  Max Deflection : Saturate  UpperLimit=30  LowerLimit=-30
  P-Depth : Gain  Gain=3
  P-Pitch : Gain  Gain=3
  PID Pitch : Selector  InputPortWidth=6  IndexOptions=Index vector (dialog)  Indices=5  OutputSizes=1
  Rate Limiter Dynamic : simulink/Discontinuities/Rate Limiter Dynamic
  dV_pid : Outport
  wires:
  Max Deflection/1 -> dV_pid/1  "dV"
  Add/1 -> Add10/2  "dV Depth (deg)"
  Add7/1 -> Derivative3/1, Integrator/1, P-Depth/1  "Erorr in z (m)"
  Zeff/1 -> Add7/2  "z (m)"
  Integrator/1 -> I-Depth/1
  P-Depth/1 -> I-Pitch4/1
  Gain36/1 -> Add9/2  "Pitch (deg)"
  Add9/1 -> Derivative/1, Integrator3/1, P-Pitch/1  "Error in Pitch (deg)"
  P-Pitch/1 -> I-Pitch3/1
  Bx/1 -> PID Pitch/1
  Derivative3/1 -> D-Depth/1
  Add1/1 -> Add10/1  "dV Pitch (deg)"
  D-Depth/1 -> I-Pitch6/1
  Derivative/1 -> D-Pitch/1
  Integrator3/1 -> I-Pitch/1
  PID Pitch/1 -> Gain36/1
  Rate Limiter Dynamic/1 -> Max Deflection/1  "dV"
  D-Pitch/1 -> I-Pitch5/1
  Target Pitch/1 -> Add9/1
  Add10/1 -> Rate Limiter Dynamic/2
  Constant/1 -> Rate Limiter Dynamic/1
  Constant1/1 -> Rate Limiter Dynamic/3
  Target Height/1 -> Add7/1
  I-Pitch/1 -> I-Pitch1/1
  I-Depth/1 -> I-Pitch2/1
  I-Pitch1/1 -> Add1/2
  I-Pitch2/1 -> Add/2
  I-Pitch3/1 -> Add1/1
  I-Pitch4/1 -> Add/1
  I-Pitch5/1 -> Add1/3
  I-Pitch6/1 -> Add/3

== system Model_6DOF_2021a/Controller/TC/n:RPS PID ==
  Target Speed : Inport
  Bv : Inport  Port=2
  Add : Sum  Inputs=+++
  Add1 : Sum  Inputs=-+
  Constant1 : Constant  Value=4
  Divide : Product  Inputs=*/
  Gain1 : Gain  Gain=14.65
  Gain4 : Gain  Gain=1.465
  Integrator : Integrator
  Rate Limiter Dynamic : simulink/Discontinuities/Rate Limiter Dynamic
  Rate Max : Constant  Value=14.65
  Rate Min : Constant  Value=-14.65
  Saturation1 : Saturate  UpperLimit=10  LowerLimit=0.01
  Selector : Selector  InputPortWidth=6  IndexOptions=Index vector (dialog)  Indices=1  OutputSizes=1
  n_ctrl : Outport  VectorParamsAs1DForOutWhenUnconnected=off
  wires:
  Saturation1/1 -> n_ctrl/1
  Selector/1 -> Add1/2  "current"
  Constant1/1 -> Divide/2
  Target Speed/1 -> Add1/1, Divide/1  "target"
  Add1/1 -> Gain1/1, Integrator/1  "error term"
  Bv/1 -> Selector/1
  Gain4/1 -> Add/3
  Gain1/1 -> Add/2
  Add/1 -> Rate Limiter Dynamic/2
  Divide/1 -> Add/1
  Rate Max/1 -> Rate Limiter Dynamic/1
  Rate Min/1 -> Rate Limiter Dynamic/3
  Integrator/1 -> Gain4/1
  Rate Limiter Dynamic/1 -> Saturation1/1

== system Model_6DOF_2021a/Controller/VZZ/dH PID ==
  Target Yaw : Inport
  Target Sway : Inport  Port=2
  Bx : Inport  Port=3
  Add1 : Sum  Inputs=+++
  Add10 : Sum
  Add2 : Sum  Inputs=+++
  Add7 : Sum  Inputs=-+
  Add9 : Sum  Inputs=-+
  Constant : Constant  Value=7.11
  Constant1 : Constant  Value=-7.11
  D-Sway : Gain  Gain=0
  D-Yaw : Gain  Gain=12.199
  Derivative : Derivative
  Derivative1 : Derivative
  Gain36 : Gain  Gain=180/pi
  I-Sway : Gain  Gain=0
  I-Yaw : Gain  Gain=0
  Integrator : Integrator
  Integrator3 : Integrator
  Max Deflection : Saturate  UpperLimit=30  LowerLimit=-30
  P-Sway1 : Gain  Gain=-1.452
  P-Yaw : Gain  Gain=3
  PID Sway : Selector  InputPortWidth=6  IndexOptions=Index vector (dialog)  Indices=2  OutputSizes=1
  PID Yaw : Selector  InputPortWidth=6  IndexOptions=Index vector (dialog)  Indices=6  OutputSizes=1
  Rate Limiter Dynamic : simulink/Discontinuities/Rate Limiter Dynamic
  dH_PID : Outport
  wires:
  Max Deflection/1 -> dH_PID/1
  Constant/1 -> Rate Limiter Dynamic/1
  Constant1/1 -> Rate Limiter Dynamic/3
  Target Yaw/1 -> Add9/1
  Add10/1 -> Rate Limiter Dynamic/2
  Derivative1/1 -> D-Yaw/1
  D-Sway/1 -> Add2/3
  P-Sway1/1 -> Add2/1
  Rate Limiter Dynamic/1 -> Max Deflection/1
  Gain36/1 -> Add9/2
  Integrator/1 -> I-Sway/1
  Add1/1 -> Add10/1
  PID Yaw/1 -> Gain36/1
  D-Yaw/1 -> Add1/3
  I-Sway/1 -> Add2/2
  Bx/1 -> PID Sway/1, PID Yaw/1
  P-Yaw/1 -> Add1/1
  PID Sway/1 -> Add7/2
  Derivative/1 -> D-Sway/1
  Target Sway/1 -> Add7/1
  Add7/1 -> Integrator/1, Derivative/1, P-Sway1/1
  I-Yaw/1 -> Add1/2
  Add2/1 -> Add10/2
  Add9/1 -> Integrator3/1, Derivative1/1, P-Yaw/1
  Integrator3/1 -> I-Yaw/1

== system Model_6DOF_2021a/Controller/VZZ/dV ==
  Bx : Inport
  Clock : Clock
  Constant4 : Constant  Value=dX_imposed
  Constant6 : Constant  Value=check_angle
  Gain1 : Gain  Gain=-1
  Gain8 : Gain  Gain=180/pi
  Integrator2 : Integrator
  MATLAB Function : MATLAB Function  TreatAsAtomicUnit=on
  Max Fin Rate : Constant  Value=7.11
  Saturation1 : Saturate  UpperLimit=20  LowerLimit=-20
  Selector2 : Selector  InputPortWidth=6  IndexOptions=Index vector (dialog)  Indices=5  OutputSizes=1
  dV_VZZ : Outport
  wires:
  Saturation1/1 -> Gain1/1, MATLAB Function/6(dVprev)
  Integrator2/1 -> Saturation1/1
  MATLAB Function/1(dVrate) -> Integrator2/1
  Gain1/1 -> dV_VZZ/1
  Bx/1 -> Selector2/1
  Selector2/1 -> Gain8/1
  Gain8/1 -> MATLAB Function/3(X5)
  Clock/1 -> MATLAB Function/2(trigger)
  Max Fin Rate/1 -> MATLAB Function/1(rate)
  Constant6/1 -> MATLAB Function/5(dXmax)
  Constant4/1 -> MATLAB Function/4(dVmax)

== system Model_6DOF_2021a/HDM/HDM B3/Effective Veloicity Calclation ==
  Bv : Inport
  uwsXi : Inport  Port=2
  uwsCG : Inport  Port=3
  Add{,1..4} (5 alike) : Sum
  Demux : Demux  Outputs=5
  Demux1 : Demux  Outputs=3
  MATLAB Function : MATLAB Function  TreatAsAtomicUnit=on
  MATLAB Function1 : MATLAB Function  TreatAsAtomicUnit=on
  MATLAB Function2 : MATLAB Function  TreatAsAtomicUnit=on
  X_SP1 : Constant  Value=[31.924; 3.861; -3.861;]
  X_SP2 : Constant  Value=[31.924; 3.861; 3.861;]
  X_SP3 : Constant  Value=[31.924; -3.861; 3.861;]
  X_SP4 : Constant  Value=[31.924; -3.861; -3.861;]
  X_XB : Constant  Value=[-10.465; 0; 9.732;]
  n1 : Constant  Value=[0; 1/sqrt(2); -1/sqrt(2);]
  n2 : Constant  Value=[0; 1/sqrt(2); 1/sqrt(2);]
  n3 : Constant  Value=[0; -1/sqrt(2); 1/sqrt(2);]
  n4 : Constant  Value=[0; -1/sqrt(2); -1/sqrt(2);]
  n5 : Constant  Value=[0; 1; 0;]
  nh : Constant  Value=[-1; 0; 0;]
  Alpha : Outport
  Beta : Outport  Port=2
  Umag : Outport  Port=3
  aXi : Outport  Port=4
  UeX : Outport  Port=5
  wires:
  Bv/1 -> MATLAB Function1/6(U_ship), MATLAB Function2/1(Bv)
  nh/1 -> MATLAB Function/1(nh)
  n1/1 -> MATLAB Function/2(n1)
  n2/1 -> MATLAB Function/3(n2)
  n3/1 -> MATLAB Function/4(n3)
  n4/1 -> MATLAB Function/5(n4)
  X_XB/1 -> MATLAB Function1/5(rXB)
  X_SP2/1 -> MATLAB Function1/2(rX2)
  X_SP3/1 -> MATLAB Function1/3(rX3)
  X_SP4/1 -> MATLAB Function1/4(rX4)
  X_SP1/1 -> MATLAB Function1/1(rX1)
  n5/1 -> MATLAB Function/6(nB)
  MATLAB Function1/1(urX1) -> Add/1
  Demux/1 -> Add/2
  Add/1 -> MATLAB Function/7(urX1)
  Add1/1 -> MATLAB Function/8(urX2)
  Add2/1 -> MATLAB Function/9(urX3)
  Add3/1 -> MATLAB Function/10(urX4)
  Add4/1 -> MATLAB Function/11(urXB)
  Demux/2 -> Add1/2
  Demux/3 -> Add2/2
  Demux/4 -> Add3/2
  Demux/5 -> Add4/2
  MATLAB Function1/5(urXB) -> Add4/1
  MATLAB Function1/4(urX4) -> Add3/1
  MATLAB Function1/3(urX3) -> Add2/1
  MATLAB Function1/2(urX2) -> Add1/1
  MATLAB Function2/2(beta) -> Beta/1
  MATLAB Function2/3(Umag) -> Umag/1
  MATLAB Function/2(UeX) -> UeX/1
  Demux1/1 -> MATLAB Function2/2(uCG)
  Demux1/2 -> MATLAB Function2/3(vCG)
  Demux1/3 -> MATLAB Function2/4(wCG)
  uwsCG/1 -> Demux1/1
  MATLAB Function2/1(alpha) -> Alpha/1
  MATLAB Function/1(aX) -> aXi/1
  uwsXi/1 -> Demux/1

== system Model_6DOF_2021a/HDM/HDM B3/Effective dX Calculation ==
  dX CTRL : Inport
  aXi : Inport  Port=2
  Add{,1..4} (5 alike) : Sum
  Demux : Demux  Outputs=5
  Demux1 : Demux  Outputs=5
  Mux6 : Mux  Inputs=5
  dXeff : Outport
  wires:
  dX CTRL/1 -> Demux/1
  aXi/1 -> Demux1/1
  Add/1 -> Mux6/1
  Add1/1 -> Mux6/2
  Add2/1 -> Mux6/3
  Add3/1 -> Mux6/4
  Add4/1 -> Mux6/5
  Demux/1 -> Add/1
  Demux/2 -> Add1/1
  Demux/3 -> Add2/1
  Demux/4 -> Add3/1
  Demux/5 -> Add4/1
  Demux1/1 -> Add/2
  Demux1/2 -> Add1/2
  Demux1/3 -> Add2/2
  Demux1/4 -> Add3/2
  Demux1/5 -> Add4/2
  Mux6/1 -> dXeff/1

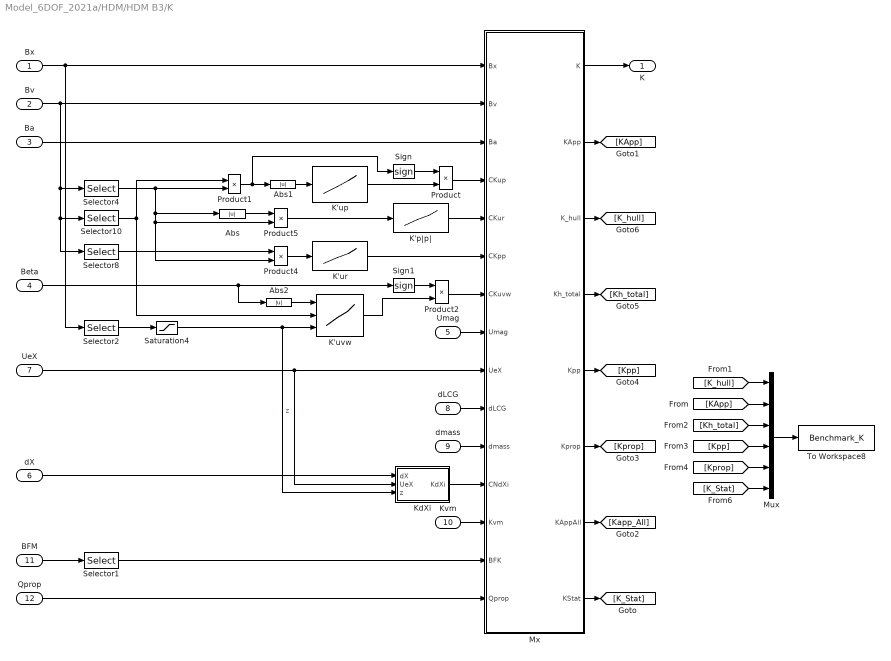
== system Model_6DOF_2021a/HDM/HDM B3/K ==
  Bx : Inport
  Bv : Inport  Port=2
  Ba : Inport  Port=3
  Beta : Inport  Port=4
  Umag : Inport  Port=5
  dX : Inport  Port=6
  UeX : Inport  Port=7
  dLCG : Inport  Port=8
  dmass : Inport  Port=9
  Kvm : Inport  Port=10
  BFM : Inport  Port=11
  Qprop : Inport  Port=12
  Abs : Abs
  Abs1 : Abs
  Abs2 : Abs
  K'p|p| : Lookup_n-D  NumberOfTableDimensions=1  BreakpointsForDimension1=|  Table=|  InternalRulePriority=Speed  RndMeth=Simplest  InputSameDT=on
      BreakpointsForDimension1=|
      | [-0.0015
      | -0.0012
      | -0.0009
      | -0.0006
      | -0.0003
      | -0.0001
      | 0.0001
      | 0.0003
      | 0.0006
      | 0.0009
      | 0.0012
      | 0.0015]
      Table=|
      | [-1.3011E-02
      | -1.6962E-02
      | -2.0682E-02
      | -3.1419E-02
      | -6.4407E-02
      | -1.9322E-01
      | 1.9322E-01
      | 6.4378E-02
      | 3.1944E-02
      | 2.1072E-02
      | 1.6415E-02
      | 1.3407E-02]
  K'up : Lookup_n-D  NumberOfTableDimensions=1  BreakpointsForDimension1=|  Table=|  InternalRulePriority=Speed  RndMeth=Simplest  InputSameDT=on
      BreakpointsForDimension1=|
      | [0.03999989
      | 0.079999993
      | 0.11999963
      | 0.15999956]
      Table=|
      | [-4.0344E-04
      | -8.1402E-04
      | -1.2116E-03
      | -1.6125E-03]
  K'ur : Lookup_n-D  NumberOfTableDimensions=1  BreakpointsForDimension1=|  Table=|  InternalRulePriority=Speed  RndMeth=Simplest  InputSameDT=on
      BreakpointsForDimension1=|
      | [-0.0015
      | -0.0012
      | -0.0009
      | -0.0006
      | -0.0003
      | -0.0001
      | 0.0001
      | 0.0003
      | 0.0006
      | 0.0009
      | 0.0012
      | 0.0015]
      Table=|
      | [-1.3011E-02
      | -1.6962E-02
      | -2.0682E-02
      | -3.1419E-02
      | -6.4407E-02
      | -1.9322E-01
      | 1.9322E-01
      | 6.4378E-02
      | 3.1944E-02
      | 2.1072E-02
      | 1.6415E-02
      | 1.3407E-02]
  K'uvw : Lookup_n-D  NumberOfTableDimensions=3  BreakpointsForDimension1=|  BreakpointsForDimension2=|  BreakpointsForDimension3=|  Table=|  InternalRulePriority=Speed  RndMeth=Simplest  InputSameDT=on
      BreakpointsForDimension1=|
      | [0
      | 4
      | 8
      | 12]
      BreakpointsForDimension2=|
      | [-5.1444E+00
      | -3.0866E+00
      | -1.5433E+00
      | ]
      Table=|
      | reshape([0.0000000E+00
      | 1.5570290E-04
      | 3.7677829E-04
      | 6.0025374E-04
      | 0.0000000E+00
      | 1.5575678E-04
      | 3.8557685E-04
      | 6.0103850E-04
      | 0.0000000E+00
      | 1.7511088E-04
      | 3.8376789E-04
      | 6.0108480E-04
      | 0.0000000E+00
      | 1.9071552E-04
      | 4.0986649E-04
      | 6.4012030E-04
      | 0.0000000E+00
      | 1.8940622E-04
      | 4.0946931E-04
      | 6.3613461E-04
      | 0.0000000E+00
      | 1.8621071E-04
      | 4.0619654E-04
      | 7.0286379E-04
      | 0.0000000E+00
      | 2.0712189E-04
      | 4.4751988E-04
      | 7.0514631E-04
      | 0.0000000E+00
      | 1.9895751E-04
      | 4.3099356E-04
      | 6.6994571E-04
      | 0.0000000E+00
      | 1.9568554E-04
      | 4.2679977E-04
      | 6.6445067E-04
      | 0.0000000E+00
      | 2.4359563E-04
      | 5.3740096E-04
      | 8.5879902E-04
      | 0.0000000E+00
      | 2.0890025E-04
      | 4.5502130E-04
      | 7.1388224E-04
      | 0.0000000E+00
      | 2.0575072E-04
      | 4.5505766E-04
      | 7.0285206E-04],[4,3,4])
      BreakpointsForDimension3=|
      | [-35.0624 -18.3724 -15.3724 -13.8724
      | ]
      settings: InputPortMap=u0,u1,u2
  KdXi : Subsystem
  Mux : Mux  Inputs=6
  Mx : MATLAB Function  TreatAsAtomicUnit=on
  Product{,1..2,4..5} (5 alike) : Product
  Saturation4 : Saturate  UpperLimit=-13.8724  LowerLimit=-35.0624
  Selector1 : Selector  InputPortWidth=6  IndexOptions=Index vector (dialog)  Indices=4  OutputSizes=1
  Selector10 : Selector  InputPortWidth=6  IndexOptions=Index vector (dialog)  Indices=1  OutputSizes=1
  Selector2 : Selector  InputPortWidth=6  IndexOptions=Index vector (dialog)  Indices=3  OutputSizes=1
  Selector4 : Selector  InputPortWidth=6  IndexOptions=Index vector (dialog)  Indices=4  OutputSizes=1
  Selector8 : Selector  InputPortWidth=6  IndexOptions=Index vector (dialog)  Indices=2  OutputSizes=1
  Sign : Signum
  Sign1 : Signum
  To Workspace8 : ToWorkspace  VariableName=Benchmark_K  SaveFormat=Timeseries  SampleTime=-1
  K : Outport
  wires:
  Bv/1 -> Selector8/1, Selector10/1, Selector4/1, Mx/2(Bv)
  Bx/1 -> Mx/1(Bx), Selector2/1
  Selector10/1 -> K'uvw/2, Product1/1
  Ba/1 -> Mx/3(Ba)
  UeX/1 -> Mx/9(UeX), KdXi/2(UeX)
  Beta/1 -> Abs2/1, Sign1/1
  Umag/1 -> Mx/8(Umag)
  dLCG/1 -> Mx/10(dLCG)
  dmass/1 -> Mx/11(dmass)
  dX/1 -> KdXi/1(dX)
  K'up/1 -> Product/2
  Product4/1 -> K'ur/1
  Selector8/1 -> Product4/1
  Abs/1 -> Product5/1
  Product5/1 -> K'p|p|/1
  Selector4/1 -> Product4/2, Product5/2, Abs/1, Product1/2
  K'ur/1 -> Mx/6(CKpp)
  KdXi/1(KdXi) -> Mx/12(CNdXi)
  Selector2/1 -> Saturation4/1
  K'uvw/1 -> Product2/2
  Product1/1 -> Sign/1, Abs1/1
  Abs1/1 -> K'up/1
  Sign/1 -> Product/1
  Product2/1 -> Mx/7(CKuvw)
  Abs2/1 -> K'uvw/1
  Mux/1 -> To Workspace8/1
  BFM/1 -> Selector1/1
  Selector1/1 -> Mx/14(BFK)
  Mx/1(K) -> K/1
  Mx/8(KStat) -> [K_Stat]
  Sign1/1 -> Product2/1
  Product/1 -> Mx/4(CKup)
  K'p|p|/1 -> Mx/5(CKur)
  Saturation4/1 -> KdXi/3(z), K'uvw/3  "z"
  Kvm/1 -> Mx/13(Kvm)
  Qprop/1 -> Mx/15(Qprop)
  Mx/2(KApp) -> [KApp]
  Mx/7(KAppAll) -> [Kapp_All]
  Mx/6(Kprop) -> [Kprop]
  Mx/5(Kpp) -> [Kpp]
  Mx/4(Kh_total) -> [Kh_total]
  Mx/3(K_hull) -> [K_hull]
  [K_hull] -> Mux/1
  [KApp] -> Mux/2
  [Kh_total] -> Mux/3
  [Kpp] -> Mux/4
  [Kprop] -> Mux/5
  [K_Stat] -> Mux/6
